simulink model "MSV_ublf"  (R2021a)
settings: Solver=ode4  StartTime=0.0  StopTime=10  FixedStep=0.001  MaxStep=0.01  RelTol=1e-3
model workspace (MAT data in the model file):
  EnableF = 1
  F_xyh = [10; 10; 1]
  GainKnownUncty = 1
  InputSat = [8591; 330.8; 839]
  InputSatOff = 1000
  Mmtx = [1  0  0; 0  1  0; 0  0  1]
  Temp = 0
  Test1 : Simulink.Parameter (value not decoded)
  boat_heading = 0
  boat_vel_x = 0
  boat_vel_y = 0
  earth_head = 2
  earth_x = 0
  earth_y = 2
  input_heading = 1
  input_x = 1
  input_y = 1
values from neighbouring files (symbols this model uses):
  Fval = [0 0 0]    [max_dist.m]    (also in test_ablf.m = [ ix iy iz ]; test_bs.m = [ ix iy iz ]; test_fxt.m = [ ix iy iz ]; test_max.m)
  LimStop = 0    [main.m]    (also in max_dist.m = 1)
libraries: dspmtrx3 x18, aerolibutil x5, simulink x1
(part 2 of 2)

== system MSV_ublf/MSV_w//uncertainty_BS/Gmatrix ==
  note: Set to 0 for G(x1) = [ 0 0 0]
  en : Inport
  x13 : Inport  Port=2
  Add g2 : Sum
  Cos : Trigonometry  Operator=cos
  Cos1 : Trigonometry  Operator=cos
  Gain : Gain  Gain=0.2
  Gain1 : Gain  Gain=0.36
  Gain2 : Gain  Gain=0.2
  Gain3 : Gain  Gain=0.36
  Matrix Concatenate : Concatenate  NumInputs=3  Mode=Multidimensional array
  Sin : Trigonometry
  Sin1 : Trigonometry
  Subtract g1 : Sum  Inputs=+-
  Switch : Switch  Criteria=u2 > Threshold
  g1 : Constant  Value=[0 0 0]'  VectorParams1D=off
  g3 : Constant  Value=0.18
  G(x1) : Outport
  wires:
  Gain2/1 -> Add g2/1
  Gain1/1 -> Subtract g1/2
  Add g2/1 -> Matrix Concatenate/2
  Sin1/1 -> Gain2/1
  x13/1 -> Cos1/1, Sin1/1, Sin/1, Cos/1
  Subtract g1/1 -> Matrix Concatenate/1
  Cos/1 -> Gain/1
  Gain/1 -> Subtract g1/1
  g3/1 -> Matrix Concatenate/3
  Sin/1 -> Gain1/1
  Gain3/1 -> Add g2/2
  Cos1/1 -> Gain3/1
  Switch/1 -> G(x1)/1
  Matrix Concatenate/1 -> Switch/1
  g1/1 -> Switch/3
  en/1 -> Switch/2

== system MSV_ublf/MSV_w//uncertainty_BS/J(η) // J (x1) ==
  note: SET = 1 FOR REVISED J(x1)
  note: Revised J(x1)
  note: Original from paper J(x1)
  note: SET = 0 FOR PAPER J(x1) [BELOW]
  Heading Angle : Inport
  Constant1 : Constant  Value=0
  Constant2 : Constant
  Constant3 : Constant  Value=0
  Constant4 : Constant
  Cos : Trigonometry  Operator=cos  OutputSignalType=real
  Cos1 : Trigonometry  Operator=cos  OutputSignalType=real
  Display : Display
  Gain1 : Gain  Gain=-1
  Gain2 : Gain  Gain=-1
  J select : Constant  Value=0
  Matrix Concatenate3 : Concatenate  NumInputs=3  Mode=Multidimensional array
  Matrix Concatenate4 : Concatenate  NumInputs=3  Mode=Multidimensional array  ConcatenateDimension=2
  Matrix Concatenate5 : Concatenate  NumInputs=3  Mode=Multidimensional array  ConcatenateDimension=2
  Matrix Concatenate6 : Concatenate  NumInputs=3  Mode=Multidimensional array  ConcatenateDimension=2
  Matrix Concatenate7 : Concatenate  NumInputs=3  Mode=Multidimensional array
  ROW 2 : Concatenate  NumInputs=3  Mode=Multidimensional array  ConcatenateDimension=2
  ROW1 : Concatenate  NumInputs=3  Mode=Multidimensional array  ConcatenateDimension=2
  ROW3 : Concatenate  NumInputs=3  Mode=Multidimensional array  ConcatenateDimension=2
  Sin : Trigonometry
  Sin1 : Trigonometry
  Switch : Switch  Criteria=u2 > Threshold
  J : Outport
  wires:
  ROW1/1 -> Matrix Concatenate3/1
  ROW 2/1 -> Matrix Concatenate3/2
  Constant2/1 -> ROW3/3
  Constant1/1 -> ROW 2/3, ROW3/2, ROW3/1, ROW1/3
  ROW3/1 -> Matrix Concatenate3/3
  Matrix Concatenate3/1 -> Switch/1
  Cos/1 -> ROW1/1, Gain1/1
  Sin/1 -> ROW1/2, ROW 2/1
  Gain1/1 -> ROW 2/2
  Cos1/1 -> Matrix Concatenate4/1, Matrix Concatenate5/2
  Matrix Concatenate6/1 -> Matrix Concatenate7/3
  Heading Angle/1 -> Cos1/1, Sin1/1, Sin/1, Cos/1
  Constant3/1 -> Matrix Concatenate4/3, Matrix Concatenate6/1, Matrix Concatenate6/2, Matrix Concatenate5/3
  Constant4/1 -> Matrix Concatenate6/3
  Matrix Concatenate5/1 -> Matrix Concatenate7/2
  Matrix Concatenate4/1 -> Matrix Concatenate7/1
  Sin1/1 -> Matrix Concatenate5/1, Gain2/1
  Switch/1 -> Display/1, J/1
  Matrix Concatenate7/1 -> Switch/3
  J select/1 -> Switch/2
  Gain2/1 -> Matrix Concatenate4/2

== system MSV_ublf/MSV_w//uncertainty_UBLF/Added Uncertainty ==
  Mdl : Inport
  Uct : Inport  Port=2
  Scope : Scope  NumInputPorts=3
  Selector : Selector  InputPortWidth=3  IndexOptions=Index vector (dialog)  Indices=1  OutputSizes=1
  Selector1 : Selector  InputPortWidth=3  IndexOptions=Index vector (dialog)  Indices=1  OutputSizes=1
  Selector2 : Selector  InputPortWidth=3  IndexOptions=Index vector (dialog)  Indices=2  OutputSizes=1
  Selector3 : Selector  InputPortWidth=3  IndexOptions=Index vector (dialog)  Indices=2  OutputSizes=1
  Selector4 : Selector  InputPortWidth=3  IndexOptions=Index vector (dialog)  Indices=3  OutputSizes=1
  Selector5 : Selector  InputPortWidth=3  IndexOptions=Index vector (dialog)  Indices=3  OutputSizes=1
  Vector Concatenate : Concatenate
  Vector Concatenate1 : Concatenate
  Vector Concatenate2 : Concatenate
  wires:
  Vector Concatenate/1 -> Scope/1
  Selector4/1 -> Vector Concatenate2/1  "mdl h"
  Selector/1 -> Vector Concatenate/1  "mdl x"
  Selector2/1 -> Vector Concatenate1/1  "mdl y"
  Vector Concatenate2/1 -> Scope/3
  Vector Concatenate1/1 -> Scope/2
  Selector1/1 -> Vector Concatenate/2  "uct x"
  Uct/1 -> Selector5/1, Selector3/1, Selector1/1
  Selector5/1 -> Vector Concatenate2/2  "uct h"
  Selector3/1 -> Vector Concatenate1/2  "uct y"
  Mdl/1 -> Selector4/1, Selector2/1, Selector/1

== system MSV_ublf/MSV_w//uncertainty_UBLF/Cmatrix ==
  x2 : Inport
  Add : Sum
  Constant : Constant  Value=0
  Gain : Gain  Gain=-24.6612
  Gain1 : Gain  Gain=25.8
  Gain2 : Gain  Gain=-25.8
  Gain3 : Gain  Gain=24.6612
  Gain4 : Gain  Gain=1.0948
  Matrix Concatenate3 : Concatenate  NumInputs=3  Mode=Multidimensional array
  Matrix Multiply : Product  Multiplication=Matrix(*)
  ROW 2 : Concatenate  NumInputs=3  Mode=Multidimensional array  ConcatenateDimension=2
  ROW1 : Concatenate  NumInputs=3  Mode=Multidimensional array  ConcatenateDimension=2
  ROW3 : Concatenate  NumInputs=3  Mode=Multidimensional array  ConcatenateDimension=2
  Row1[x2] : dspmtrx3/Submatrix  RowSpan=One row  RowStartMode=First  RowStartIndex=1  RowEndMode=Last  RowEndIndex=1  ColSpan=One column  ColStartMode=First  ColStartIndex=1  ColEndMode=Last  ColEndIndex=1
  Row2[x2] : dspmtrx3/Submatrix  RowSpan=One row  RowStartMode=Middle  RowStartIndex=1  RowEndMode=Last  RowEndIndex=1  ColSpan=One column  ColStartMode=First  ColStartIndex=1  ColEndMode=Last  ColEndIndex=1
  Row3[x2] : dspmtrx3/Submatrix  RowSpan=One row  RowStartMode=Last  RowStartIndex=1  RowEndMode=Last  RowEndIndex=1  ColSpan=One column  ColStartMode=First  ColStartIndex=1  ColEndMode=Last  ColEndIndex=1
  C(x2)x2 : Outport
  wires:
  ROW1/1 -> Matrix Concatenate3/1
  ROW 2/1 -> Matrix Concatenate3/2
  ROW3/1 -> Matrix Concatenate3/3
  Constant/1 -> ROW3/3, ROW 2/2, ROW 2/1, ROW1/2, ROW1/1
  Row1[x2]/1 -> Gain2/1, Gain1/1  "x_vel"
  Matrix Concatenate3/1 -> Matrix Multiply/1  "C(x2)"
  Gain/1 -> ROW1/3
  Gain1/1 -> ROW 2/3
  Gain2/1 -> ROW3/2
  Gain3/1 -> Add/1
  Row2[x2]/1 -> Gain/1, Gain3/1  "y_vel"
  Gain4/1 -> Add/2
  Add/1 -> ROW3/1
  Row3[x2]/1 -> Gain4/1  "ang_vel"
  x2/1 -> Matrix Multiply/2, Row3[x2]/1, Row1[x2]/1, Row2[x2]/1  "x2"
  Matrix Multiply/1 -> C(x2)x2/1

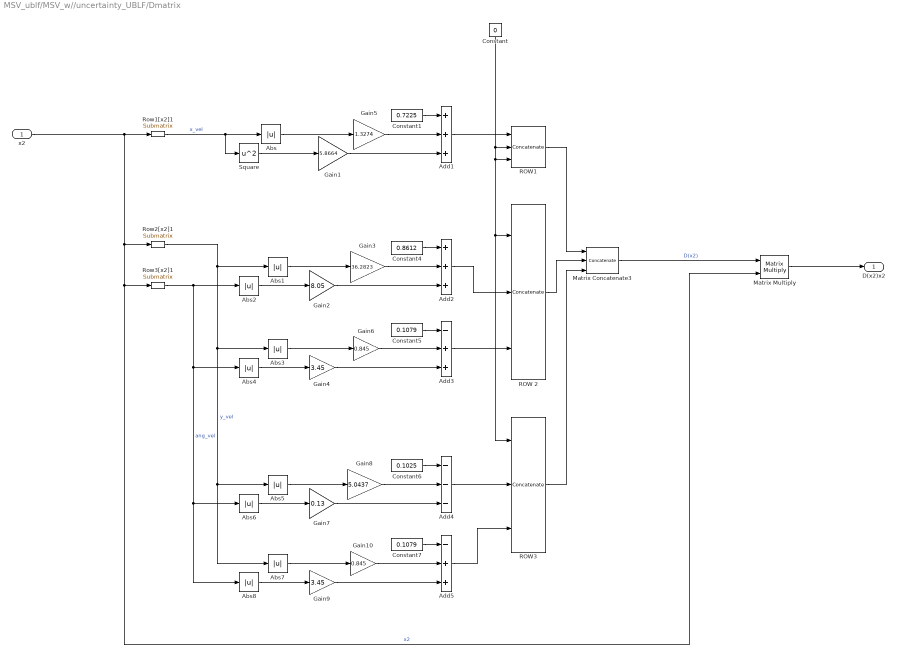
== system MSV_ublf/MSV_w//uncertainty_UBLF/Dmatrix ==
  x2 : Inport
  Abs{,1..8} (9 alike) : Abs
  Add1 : Sum  Inputs=+++
  Add2 : Sum  Inputs=+++
  Add3 : Sum  Inputs=-++
  Add4 : Sum  Inputs=---
  Add5 : Sum  Inputs=-++
  Constant : Constant  Value=0
  Constant1 : Constant  Value=0.7225
  Constant4 : Constant  Value=0.8612
  Constant5 : Constant  Value=0.1079
  Constant6 : Constant  Value=0.1025
  Constant7 : Constant  Value=0.1079
  Gain1 : Gain  Gain=5.8664
  Gain10 : Gain  Gain=0.845
  Gain2 : Gain  Gain=8.05
  Gain3 : Gain  Gain=36.2823
  Gain4 : Gain  Gain=3.45
  Gain5 : Gain  Gain=1.3274
  Gain6 : Gain  Gain=0.845
  Gain7 : Gain  Gain=0.13
  Gain8 : Gain  Gain=5.0437
  Gain9 : Gain  Gain=3.45
  Matrix Concatenate3 : Concatenate  NumInputs=3  Mode=Multidimensional array
  Matrix Multiply : Product  Multiplication=Matrix(*)
  ROW 2 : Concatenate  NumInputs=3  Mode=Multidimensional array  ConcatenateDimension=2
  ROW1 : Concatenate  NumInputs=3  Mode=Multidimensional array  ConcatenateDimension=2
  ROW3 : Concatenate  NumInputs=3  Mode=Multidimensional array  ConcatenateDimension=2
  Row1[x2]1 : dspmtrx3/Submatrix  RowSpan=One row  RowStartMode=First  RowStartIndex=1  RowEndMode=Last  RowEndIndex=1  ColSpan=One column  ColStartMode=First  ColStartIndex=1  ColEndMode=Last  ColEndIndex=1
  Row2[x2]1 : dspmtrx3/Submatrix  RowSpan=One row  RowStartMode=Middle  RowStartIndex=1  RowEndMode=Last  RowEndIndex=1  ColSpan=One column  ColStartMode=First  ColStartIndex=1  ColEndMode=Last  ColEndIndex=1
  Row3[x2]1 : dspmtrx3/Submatrix  RowSpan=One row  RowStartMode=Last  RowStartIndex=1  RowEndMode=Last  RowEndIndex=1  ColSpan=One column  ColStartMode=First  ColStartIndex=1  ColEndMode=Last  ColEndIndex=1
  Square : Math  Operator=square  SaturateOnIntegerOverflow=on
  D(x2)x2 : Outport
  wires:
  Constant/1 -> ROW 2/1, ROW3/1, ROW1/3, ROW1/2
  ROW3/1 -> Matrix Concatenate3/3
  ROW 2/1 -> Matrix Concatenate3/2
  ROW1/1 -> Matrix Concatenate3/1
  Constant1/1 -> Add1/1
  Gain5/1 -> Add1/2
  Gain1/1 -> Add1/3
  Abs/1 -> Gain5/1
  Square/1 -> Gain1/1
  Row1[x2]1/1 -> Abs/1, Square/1  "x_vel"
  Add1/1 -> ROW1/1
  Matrix Concatenate3/1 -> Matrix Multiply/1  "D(x2)"
  Abs1/1 -> Gain3/1
  Gain2/1 -> Add2/3
  Gain3/1 -> Add2/2
  Constant4/1 -> Add2/1
  Add2/1 -> ROW 2/2
  Abs2/1 -> Gain2/1
  Abs4/1 -> Gain4/1
  Constant5/1 -> Add3/1
  Gain6/1 -> Add3/2
  Gain4/1 -> Add3/3
  Abs3/1 -> Gain6/1
  Add3/1 -> ROW 2/3
  Row3[x2]1/1 -> Abs8/1, Abs6/1, Abs4/1, Abs2/1  "ang_vel"
  Abs7/1 -> Gain10/1
  Gain9/1 -> Add5/3
  Gain10/1 -> Add5/2
  Constant7/1 -> Add5/1
  Abs8/1 -> Gain9/1
  Row2[x2]1/1 -> Abs7/1, Abs5/1, Abs3/1, Abs1/1  "y_vel"
  Abs6/1 -> Gain7/1
  Constant6/1 -> Add4/1
  Gain8/1 -> Add4/2
  Gain7/1 -> Add4/3
  Abs5/1 -> Gain8/1
  Add4/1 -> ROW3/2
  Add5/1 -> ROW3/3
  x2/1 -> Matrix Multiply/2, Row3[x2]1/1, Row2[x2]1/1, Row1[x2]1/1  "x2"
  Matrix Multiply/1 -> D(x2)x2/1

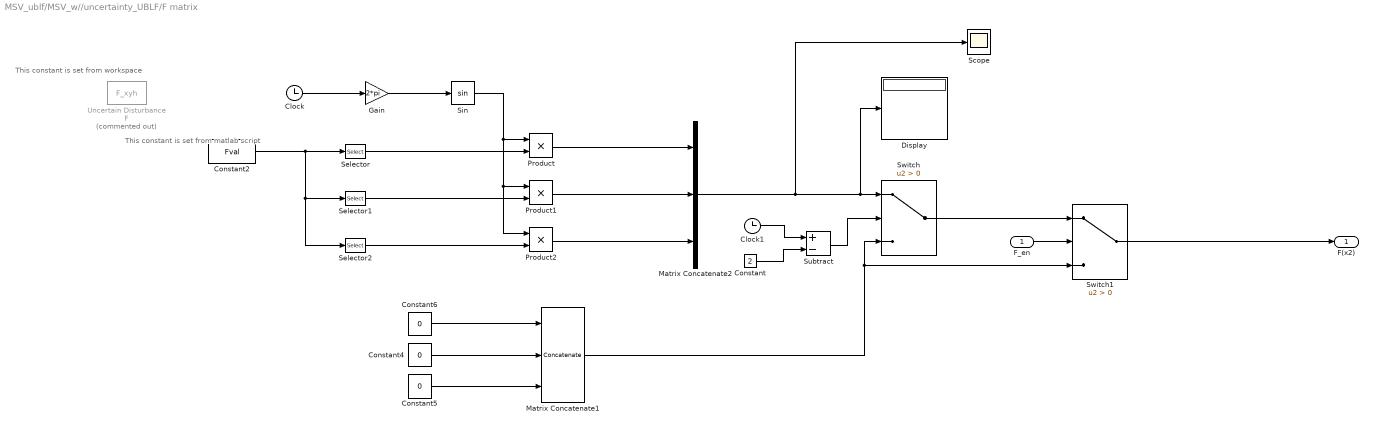
== system MSV_ublf/MSV_w//uncertainty_UBLF/F matrix ==
  note: This constant is set from matlab script
  note: This constant is set from workspace
  F_en : Inport
  Clock : Clock
  Clock1 : Clock
  Constant : Constant  Value=2
  Constant2 : Constant  Value=Fval
  Constant4 : Constant  Value=0
  Constant5 : Constant  Value=0
  Constant6 : Constant  Value=0
  Display : Display
  Gain : Gain  Gain=2*pi
  Matrix Concatenate1 : Concatenate  NumInputs=3  Mode=Multidimensional array
  Matrix Concatenate2 : Concatenate  NumInputs=3  Mode=Multidimensional array
  Product : Product
  Product1 : Product
  Product2 : Product
  Scope : Scope
  Selector : Selector  InputPortWidth=3  IndexOptions=Index vector (dialog)  Indices=1  OutputSizes=1
  Selector1 : Selector  InputPortWidth=3  IndexOptions=Index vector (dialog)  Indices=2  OutputSizes=1
  Selector2 : Selector  InputPortWidth=3  IndexOptions=Index vector (dialog)  Indices=3  OutputSizes=1
  Sin : Trigonometry
  Subtract : Sum  Inputs=+-
  Switch : Switch  Criteria=u2 > Threshold
  Switch1 : Switch  Criteria=u2 > Threshold
  Uncertain Disturbance F : Constant  Commented=on  Value=F_xyh
  F(x2) : Outport
  wires:
  F_en/1 -> Switch1/2
  Switch1/1 -> F(x2)/1
  Constant5/1 -> Matrix Concatenate1/3
  Constant4/1 -> Matrix Concatenate1/2
  Constant6/1 -> Matrix Concatenate1/1
  Matrix Concatenate1/1 -> Switch1/3, Switch/3
  Matrix Concatenate2/1 -> Scope/1, Display/1, Switch/1
  Clock1/1 -> Subtract/1
  Constant/1 -> Subtract/2
  Subtract/1 -> Switch/2
  Switch/1 -> Switch1/1
  Product/1 -> Matrix Concatenate2/1
  Product2/1 -> Matrix Concatenate2/3
  Product1/1 -> Matrix Concatenate2/2
  Sin/1 -> Product1/1, Product2/1, Product/1
  Selector/1 -> Product/2
  Selector1/1 -> Product1/2
  Selector2/1 -> Product2/2
  Gain/1 -> Sin/1
  Clock/1 -> Gain/1
  Constant2/1 -> Selector2/1, Selector1/1, Selector/1

== system MSV_ublf/MSV_w//uncertainty_UBLF/Gmatrix ==
  note: Set to 0 for G(x1) = [ 0 0 0]
  en : Inport
  x13 : Inport  Port=2
  Add g2 : Sum
  Cos : Trigonometry  Operator=cos
  Cos1 : Trigonometry  Operator=cos
  Gain : Gain  Gain=0.2
  Gain1 : Gain  Gain=0.36
  Gain2 : Gain  Gain=0.2
  Gain3 : Gain  Gain=0.36
  Matrix Concatenate : Concatenate  NumInputs=3  Mode=Multidimensional array
  Sin : Trigonometry
  Sin1 : Trigonometry
  Subtract g1 : Sum  Inputs=+-
  Switch : Switch  Criteria=u2 > Threshold
  g1 : Constant  Value=[0 0 0]'  VectorParams1D=off
  g3 : Constant  Value=0.18
  G(x1) : Outport
  wires:
  Gain2/1 -> Add g2/1
  Gain1/1 -> Subtract g1/2
  Add g2/1 -> Matrix Concatenate/2
  Sin1/1 -> Gain2/1
  x13/1 -> Cos1/1, Sin1/1, Sin/1, Cos/1
  Subtract g1/1 -> Matrix Concatenate/1
  Cos/1 -> Gain/1
  Gain/1 -> Subtract g1/1
  g3/1 -> Matrix Concatenate/3
  Sin/1 -> Gain1/1
  Gain3/1 -> Add g2/2
  Cos1/1 -> Gain3/1
  Switch/1 -> G(x1)/1
  Matrix Concatenate/1 -> Switch/1
  g1/1 -> Switch/3
  en/1 -> Switch/2

== system MSV_ublf/MSV_w//uncertainty_UBLF/J(η) // J (x1) ==
  note: SET = 1 FOR REVISED J(x1)
  note: Revised J(x1)
  note: Original from paper J(x1)
  note: SET = 0 FOR PAPER J(x1) [BELOW]
  Heading Angle : Inport
  Constant1 : Constant  Value=0
  Constant2 : Constant
  Constant3 : Constant  Value=0
  Constant4 : Constant
  Cos : Trigonometry  Operator=cos  OutputSignalType=real
  Cos1 : Trigonometry  Operator=cos  OutputSignalType=real
  Display : Display
  Gain1 : Gain  Gain=-1
  Gain2 : Gain  Gain=-1
  J select : Constant  Value=0
  Matrix Concatenate3 : Concatenate  NumInputs=3  Mode=Multidimensional array
  Matrix Concatenate4 : Concatenate  NumInputs=3  Mode=Multidimensional array  ConcatenateDimension=2
  Matrix Concatenate5 : Concatenate  NumInputs=3  Mode=Multidimensional array  ConcatenateDimension=2
  Matrix Concatenate6 : Concatenate  NumInputs=3  Mode=Multidimensional array  ConcatenateDimension=2
  Matrix Concatenate7 : Concatenate  NumInputs=3  Mode=Multidimensional array
  ROW 2 : Concatenate  NumInputs=3  Mode=Multidimensional array  ConcatenateDimension=2
  ROW1 : Concatenate  NumInputs=3  Mode=Multidimensional array  ConcatenateDimension=2
  ROW3 : Concatenate  NumInputs=3  Mode=Multidimensional array  ConcatenateDimension=2
  Sin : Trigonometry
  Sin1 : Trigonometry
  Switch : Switch  Criteria=u2 > Threshold
  J : Outport
  wires:
  ROW1/1 -> Matrix Concatenate3/1
  ROW 2/1 -> Matrix Concatenate3/2
  Constant2/1 -> ROW3/3
  Constant1/1 -> ROW 2/3, ROW3/2, ROW3/1, ROW1/3
  ROW3/1 -> Matrix Concatenate3/3
  Matrix Concatenate3/1 -> Switch/1
  Cos/1 -> ROW1/1, Gain1/1
  Sin/1 -> ROW1/2, ROW 2/1
  Gain1/1 -> ROW 2/2
  Cos1/1 -> Matrix Concatenate4/1, Matrix Concatenate5/2
  Matrix Concatenate6/1 -> Matrix Concatenate7/3
  Heading Angle/1 -> Cos1/1, Sin1/1, Sin/1, Cos/1
  Constant3/1 -> Matrix Concatenate4/3, Matrix Concatenate6/1, Matrix Concatenate6/2, Matrix Concatenate5/3
  Constant4/1 -> Matrix Concatenate6/3
  Matrix Concatenate5/1 -> Matrix Concatenate7/2
  Matrix Concatenate4/1 -> Matrix Concatenate7/1
  Sin1/1 -> Matrix Concatenate5/1, Gain2/1
  Switch/1 -> Display/1, J/1
  Matrix Concatenate7/1 -> Switch/3
  J select/1 -> Switch/2
  Gain2/1 -> Matrix Concatenate4/2

== matlab function MSV_ublf/Backstepping Control/MATLAB Function ==
  settings: updateMethod=DISCRETE
  data: CDG input; u output; x_Err output; y_Err output; h_Err output; M input; J input; X1 input; X2 input; X1d input; unused input; unused1 input size=1; test1 output; test2 output
function [u, x_Err, y_Err, h_Err, test1, test2] =  fcn( CDG, M, J ,X1, X2, X1d, ~, ~)
    
    tstep   = 0.001;
    
    persistent last_alpha1 
    if isempty(last_alpha1) 
        last_alpha1=X2;
    end
    
    persistent last_X1d 
    if isempty(last_X1d) 
        last_X1d=X1d;
    end
    
    X1d_dot = (X1d - last_X1d)/tstep;
    last_X1d = X1d;

    JT      = J';    % Transpose jacobian

    
    % Set Gain Values
    K1      = 30 ; % 100*[ 0.01 ; 0.01 ; 0.01 ];           % Gains used with ALPHA1    ### NOTE SET MUCH HIGHER THAN VALUES IN PAPER ####
    K2      = 200; %5*[ 20 0 0 ; 0 20 0 ; 0 0 20 ];     % Gains used with u          ### NOTE SET MUCH HIGHER THAN VALUES IN PAPER ####
    

% ### STEP 1 ###
    
    Z1      = X1 - X1d;          % Z1 position/hdg error
    
    %ALPHA 1

    ALPHA1  = JT*(X1d_dot - Z1.*K1 );
    
    A1_dot = (ALPHA1-last_alpha1)/tstep;
    last_alpha1 = ALPHA1;
    
% ### STEP 2 ###

    Z2      = X2 - ALPHA1;  % Z2 velocity error
    CTRL    = -CDG - J*Z1 - K2.*Z2 + M*A1_dot;
    
% Function Outputs

u       = CTRL;
x_Err   = 0;
y_Err   = 0;
h_Err   = 0;
test1   = 0;
test2   = Z1;

== matlab function MSV_ublf/FxT uBLF_v1.1/SymUBLF1 ==
  settings: updateMethod=DISCRETE
  data: F2 input; G2 input; G1 input; X1 input; X2 input; Xd input; unused input; unused1 input; u output; xErr output; yErr output; hErr output; test1 output
function [u,xErr, yErr, hErr, test1 ] = fcn(F2, G2, G1, X1, X2, Xd, ~, ~)

    %Simulation settings
    tstep = 0.001;
    
    % Set persistent variables for derivatives
    persistent last_x1d
    if isempty (last_x1d)
        last_x1d = Xd;
    end
    
    persistent last_A1
    if isempty(last_A1)
        last_A1 = X2;
    end
    
    % K (3x1) Barrier limits
    K       = 5*[ 0.005
                0.005
                0.005 ]; 

    % fixed time parameters (a/b maybe should be vectors?)
      
    a1      = 5;
    b1      = 1;
    a2      = 5;
    b2      = 1;

    eps10   = 0.00001;
    eps20   = 0.00001;
    
    eps1    = 0.00008;
    eps2    = 0.00001;

% ### STEP 1 ####

    % Z1 (3x1) - Position error
    Z1      = X1 - Xd;
    
    % ETA (3x1)
    ETA     = ((K.^2).*Z1) ./ ( (K.^2)-(Z1.^2)); 
    nETA    = norm(ETA); %mETA    = sqrt(sum(ETA.^2)); % magnitude of ETA vector for S1 switched term ¦ changed to norm(ETA) ?
    
    % OMEGA (3x1)
    OMEGA   = ( (K.^2).*( (K.^2)+(Z1.^2) ) ) ./ ( ( (K.^2)-(Z1.^2) ).^2 ) ;

    % Switched Term 1st step S1
    if nETA < eps10
        %test%S1 = ( (ETA.^2).^(3/4)); 
        S1 = (5/4)*(ETA' * ETA)*((eps10^2)^(-1/4)) +  (-1/4)*((ETA' * ETA)^2)*((eps10^2)^(-5/4)) ;
    else
       S1 = ( (ETA' * ETA)^(3/4));        
    end
    
    % X1 derivative used in ALPHA1
    Xd_dot = (Xd - last_x1d)/tstep;
    last_x1d = Xd;
    
    % Calculate ALPHA1 virtual control for step 2
    ALPHA1_HAT  = -(OMEGA.*Xd_dot) +  ( (0.5^(3/4))*a1 )*( (ETA/(ETA' * ETA))*S1 ) + ((0.5^2)*b1)*((ETA*(ETA' * ETA))) ;
    ALPHA1_BAR  = diag([1/OMEGA(1) 1/OMEGA(2) 1/OMEGA(3)])*ALPHA1_HAT;
    nA1B        = norm(ALPHA1_BAR);
    ETA_OMEGA   = ETA .* OMEGA;
    nETA_OMEGA  = norm(ETA_OMEGA);
    g1          = inv(G1);
    
    ALPHA1      = -g1 * (  (ETA_OMEGA*((nA1B)^2) ) / ( sqrt( ( (nETA_OMEGA)^2 ) * ( (nA1B)^2 ) + eps1^2 ) )  );
    
% ### STEP 2 ###

    %Z2 = X2 - ALPHA1
    Z2      = X2 - ALPHA1;
    nZ2     = norm(Z2);   % norm of vector Z2 used to select S2 term below
    
    % Switched Term 2nd step S2
    if nZ2 < eps20
        %test S2 = ( (Z2.^2).^(3/4));
        S2 = (5/4)*(Z2' * Z2)*((eps20^2)^(-1/4)) +  (-1/4)*((Z2' * Z2).^2)*((eps20^2)^(-5/4)) ;
    else
       S2 = ( (Z2' * Z2)^(3/4));        
    end
    
    % ALPHA1 derivative used in ALPHA2_HAT
    A1_dot = (ALPHA1 - last_A1)/tstep;
    last_A1 = ALPHA1;    
    
    % Calculate control signal
    AH2_A       = ( (0.5^(3/4))*a2 )*( (Z2 / (Z2' * Z2))*S2 );
    AH2_B       = ( (0.5^2)*b2) * ((Z2*(Z2' * Z2)           ));
    ALPHA2_HAT  = ( -(A1_dot) + AH2_A + AH2_B );
    g2          = inv(G2);
    CTRL        = -g2 * ( (Z2 .* (ALPHA2_HAT.^2)) ./ ( sqrt (((Z2.^2).*(ALPHA2_HAT.^2) + eps2^2)) ) + (G1 * ETA_OMEGA) +F2 );      

%Function outputs
xErr    = [Z1(1) ; K(1) ; -K(1)];   % error and BLF limits
yErr    = [Z1(2) ; K(2) ; -K(2)];   % error and BLF limits
hErr    = [Z1(3) ; K(3) ; -K(3)];   % error and BLF limits
test1   = 0;                        % test output
u       = CTRL;


%%[2022.02.23.Wed] Changed Functions from v1.2(correcting for elementwise to matrix functions)

%     % Switched Term 1st step S1
%     if mETA < eps10
%         %test%S1 = ( (ETA.^2).^(3/4)); 
%         S1 = (5/4)*(ETA.^2)*((eps10^2)^(-1/4)) +  (-1/4)*((ETA.^2).^2)*((eps10^2)^(-5/4)) ;
%     else
%        S1 = ( (ETA.^2).^(3/4));        
%     end

%     % Calculate ALPHA1 virtual control for step 2
%     ALPHA1_HAT  = -(OMEGA.*Xd_dot) + ( ((0.5^(3/4)).*a1).*((ETA ./ (ETA.^2)).*S1) ) + ( ((0.5^2).*b1).*((ETA.*(ETA.^2))) );
%     ALPHA1_BAR  = diag([1/OMEGA(1) 1/OMEGA(2) 1/OMEGA(3)])*ALPHA1_HAT;
%     nA1B        = norm(ALPHA1_BAR);
%     ETA_OMEGA   = ETA .* OMEGA;
%     nETA_OMEGA  = norm(ETA_OMEGA);
%     g1          = inv(G1);

    % wrong sqrt in denom of ALPHA1 below
%   ALPHA1      = -g1 * (( ETA_OMEGA*((nA1B)^2) ) ./ (sqrt( (nETA_OMEGA)^2)*((nA1B)^2) + eps1^2  ));

== matlab function MSV_ublf/FxT uBLF_v1.4/SymUBLF1 ==
  settings: updateMethod=DISCRETE
  data: F2 input; G2 input; G1 input; X1 input; X2 input; Xd input; unused input; unused1 input; u output; xErr output; yErr output; hErr output; test1 output
function [u,xErr, yErr, hErr, test1 ] = fcn(F2, G2, G1, X1, X2, Xd, ~, ~)

    %Simulation settings
    tstep = 0.001;
    
    % Set persistent variables for derivatives
    persistent last_x1d
    if isempty (last_x1d)
        last_x1d = Xd;
    end
    
    persistent last_A1
    if isempty(last_A1)
        last_A1 = X2;
    end
    
    % K (3x1) Barrier limits
    K       = 5*[ 0.005
                0.005
                0.005 ]; 

    % fixed time parameters (a/b maybe should be vectors?)
      
    a1      = 5;
    b1      = 1;
    a2      = 5;
    b2      = 1;

    eps10   = 0.00001;
    eps20   = 0.00001;
    
    eps1    = 0.00008;
    eps2    = 0.00001;

% ### STEP 1 ####

    % Z1 (3x1) - Position error
    Z1      = X1 - Xd;
    
    % ETA (3x1)
    ETA     = ((K.^2).*Z1) ./ ( (K.^2)-(Z1.^2)); 
    nETA    = norm(ETA); %mETA    = sqrt(sum(ETA.^2)); % magnitude of ETA vector for S1 switched term ¦ changed to norm(ETA) ?
    
    % OMEGA (3x1)
    OMEGA   = ( (K.^2).*( (K.^2)+(Z1.^2) ) ) ./ ( ( (K.^2)-(Z1.^2) ).^2 ) ;

    % Switched Term 1st step S1
    if nETA < eps10
        %test%S1 = ( (ETA.^2).^(3/4)); 
        S1 = (5/4)*(ETA' * ETA)*((eps10^2)^(-1/4)) +  (-1/4)*((ETA' * ETA)^2)*((eps10^2)^(-5/4)) ;
    else
       S1 = ( (ETA' * ETA)^(3/4));        
    end
    
    % X1 derivative used in ALPHA1
    Xd_dot = (Xd - last_x1d)/tstep;
    last_x1d = Xd;
    
    % Calculate ALPHA1 virtual control for step 2
    ALPHA1_HAT  = -(OMEGA.*Xd_dot) +  ( (0.5^(3/4))*a1 )*( (ETA/(ETA' * ETA))*S1 ) + ((0.5^2)*b1)*((ETA*(ETA' * ETA))) ;
    ALPHA1_BAR  = diag([1/OMEGA(1) 1/OMEGA(2) 1/OMEGA(3)])*ALPHA1_HAT;
    nA1B        = norm(ALPHA1_BAR);
    ETA_OMEGA   = ETA .* OMEGA;
    nETA_OMEGA  = norm(ETA_OMEGA);
    g1          = inv(G1);
    
    ALPHA1      = -g1 * (  (ETA_OMEGA*((nA1B)^2) ) / ( sqrt( ( (nETA_OMEGA)^2 ) * ( (nA1B)^2 ) + eps1^2 ) )  );
    
% ### STEP 2 ###

    %Z2 = X2 - ALPHA1
    Z2      = X2 - ALPHA1;
    nZ2     = norm(Z2);   % norm of vector Z2 used to select S2 term below
    
    % Switched Term 2nd step S2
    if nZ2 < eps20
        %test S2 = ( (Z2.^2).^(3/4));
        S2 = (5/4)*(Z2' * Z2)*((eps20^2)^(-1/4)) +  (-1/4)*((Z2' * Z2).^2)*((eps20^2)^(-5/4)) ;
    else
       S2 = ( (Z2' * Z2)^(3/4));        
    end
    
    % ALPHA1 derivative used in ALPHA2_HAT
    A1_dot = (ALPHA1 - last_A1)/tstep;
    last_A1 = ALPHA1;    
    
    % Calculate control signal
    AH2_A       = ( (0.5^(3/4))*a2 )*( (Z2 / (Z2' * Z2))*S2 );
    AH2_B       = ( (0.5^2)*b2) * ((Z2*(Z2' * Z2)           ));
    ALPHA2_HAT  = ( -(A1_dot) + AH2_A + AH2_B );
    g2          = inv(G2);
    CTRL        = -g2 * ( (Z2 .* (ALPHA2_HAT.^2)) ./ ( sqrt (((Z2.^2).*(ALPHA2_HAT.^2) + eps2^2)) ) + (G1 * ETA_OMEGA) +F2 );      

%Function outputs
xErr    = [Z1(1) ; K(1) ; -K(1)];   % error and BLF limits
yErr    = [Z1(2) ; K(2) ; -K(2)];   % error and BLF limits
hErr    = [Z1(3) ; K(3) ; -K(3)];   % error and BLF limits
test1   = 0;                        % test output
u       = CTRL;


%%[2022.02.23.Wed] Changed Functions from v1.2(correcting for elementwise to matrix functions)

%     % Switched Term 1st step S1
%     if mETA < eps10
%         %test%S1 = ( (ETA.^2).^(3/4)); 
%         S1 = (5/4)*(ETA.^2)*((eps10^2)^(-1/4)) +  (-1/4)*((ETA.^2).^2)*((eps10^2)^(-5/4)) ;
%     else
%        S1 = ( (ETA.^2).^(3/4));        
%     end

%     % Calculate ALPHA1 virtual control for step 2
%     ALPHA1_HAT  = -(OMEGA.*Xd_dot) + ( ((0.5^(3/4)).*a1).*((ETA ./ (ETA.^2)).*S1) ) + ( ((0.5^2).*b1).*((ETA.*(ETA.^2))) );
%     ALPHA1_BAR  = diag([1/OMEGA(1) 1/OMEGA(2) 1/OMEGA(3)])*ALPHA1_HAT;
%     nA1B        = norm(ALPHA1_BAR);
%     ETA_OMEGA   = ETA .* OMEGA;
%     nETA_OMEGA  = norm(ETA_OMEGA);
%     g1          = inv(G1);

    % wrong sqrt in denom of ALPHA1 below
%   ALPHA1      = -g1 * (( ETA_OMEGA*((nA1B)^2) ) ./ (sqrt( (nETA_OMEGA)^2)*((nA1B)^2) + eps1^2  ));

== matlab function MSV_ublf/FxT uBLF_v1.1/UBLF ==
  settings: updateMethod=DISCRETE
  data: F2 input; G2 input; G1 input; X1 input; X2 input; Xd input; unused input; unused1 input; u output; xErr output; yErr output; hErr output; test1 output; test2 output
function [u,xErr, yErr, hErr, test1, test2 ] = fcn(F2, G2, G1, X1, X2, Xd, ~, ~)

    %Simulation settings
    tstep = 0.001;
    
    % Set persistent variables for derivatives
    persistent last_x1d
    if isempty (last_x1d)
        last_x1d = Xd;
    end
    
    persistent last_A1
    if isempty(last_A1)
        last_A1 = X2;
    end
    
    % Barrier limits
    % Lower Limit (-KL)
    KL      = 1*[   0.008
                    0.005
                    0.006 ];       
    % Higher/Upper Limit (KH)
    KH      = 1*[   0.016
                    0.015
                    0.011 ]; 
    % fixed time parameterS
      
    a1      = 2*5;
    b1      = 30;
    a2      = 2*5;
    b2      = 30;

    eps10   = 0.0001;
    eps20   = 0.0001;
    
    eps1    = 0.00005;
    eps2    = eps1;
    
    kpa1 = min(a1,a2);
    kpa2 = min(b1,b2);
    
    tmax = 5.867/kpa1 + 1/kpa2;

% ### STEP 1 ####

    % Z1 (3x1) - Position error
    Z1      = X1 - Xd;
    
    % ETA (3x1)
    ETA     = ( (KH .* KL).*Z1 ) ./ ( (KH - Z1) .* (KL + Z1) ) ; 
    nETA    = norm(ETA); %mETA    = sqrt(sum(ETA.^2)); % magnitude of ETA vector for S1 switched term ¦ changed to norm(ETA) ?
    
    % OMEGA (3x1)
    OMEGA   = ( KH .* KL .*(KH .* KL + Z1.^2 ) ) ./ ( (KH - Z1).^2  .* (KL + Z1).^2 ) ;

    % Switched Term 1st step S1
    if nETA < eps10
        %test%S1 = ( (ETA.^2).^(3/4)); 
        S1 = (5/4)*(ETA' * ETA)*((eps10^2)^(-1/4)) +  (-1/4)*((ETA' * ETA)^2)*((eps10^2)^(-5/4)) ;
    else
       S1 = ( (ETA' * ETA)^(3/4));        
    end
    
    % X1 derivative used in ALPHA1
    Xd_dot = (Xd - last_x1d)/tstep;
    last_x1d = Xd;
    
    % Calculate ALPHA1 virtual control for step 2
    ALPHA1_HAT  = -(OMEGA.*Xd_dot) +  ( (0.5^(3/4))*a1 )*( (ETA/(ETA' * ETA))*S1 ) + ((0.5^2)*b1)*((ETA*(ETA' * ETA))) ;
    ALPHA1_BAR  = diag([1/OMEGA(1) 1/OMEGA(2) 1/OMEGA(3)])*ALPHA1_HAT;
    nA1B        = norm(ALPHA1_BAR);
    ETA_OMEGA   = ETA .* OMEGA;
    nETA_OMEGA  = norm(ETA_OMEGA);
    g1          = G1';
    
    ALPHA1      = -g1 * (  (ETA_OMEGA*((nA1B)^2) ) / ( sqrt( ( (nETA_OMEGA)^2 ) * ( (nA1B)^2 ) + eps1^2 ) )  );
    
% ### STEP 2 ###

    %Z2 = X2 - ALPHA1
    Z2      = X2 - ALPHA1;
    nZ2     = norm(Z2);   % norm of vector Z2 used to select S2 term below
    
    % Switched Term 2nd step S2
    if nZ2 < eps20
        %test S2 = ( (Z2.^2).^(3/4));
        S2 = (5/4)*(Z2' * Z2)*((eps20^2)^(-1/4)) +  (-1/4)*((Z2' * Z2).^2)*((eps20^2)^(-5/4)) ;
    else
       S2 = ( (Z2' * Z2)^(3/4));        
    end
    
    % ALPHA1 derivative used in ALPHA2_HAT
    A1_dot = (ALPHA1 - last_A1)/tstep;
    last_A1 = ALPHA1;    
    
    % Calculate control signal
    AH2_A       = ( (0.5^(3/4))*a2 )*( (Z2 / (Z2' * Z2))*S2 );
    AH2_B       = ( (0.5^2)*b2) * ((Z2*(Z2' * Z2)           ));
    ALPHA2_HAT  = ( -(A1_dot) + AH2_A + AH2_B );
    g2          = inv(G2);
    CTRL        = -g2 * ( (Z2 .* (ALPHA2_HAT.^2)) ./ ( sqrt (((Z2.^2).*(ALPHA2_HAT.^2) + eps2^2)) ) + (Z2/(Z2'*Z2))*ETA_OMEGA'*g1*Z2 + F2 );
%   CTRL        = -g2 * ( (Z2 .* (ALPHA2_HAT.^2)) ./ ( sqrt (((Z2.^2).*(ALPHA2_HAT.^2) + eps2^2)) ) + (G1 * ETA_OMEGA) +F2 );  

%Function outputs
xErr    = [Z1(1) ; KH(1) ; -KL(1)];   % error and BLF limits
yErr    = [Z1(2) ; KH(2) ; -KL(2)];   % error and BLF limits
hErr    = [Z1(3) ; KH(3) ; -KL(3)];   % error and BLF limits
test1   = Z1 ;                        % test output
test2   = [tmax, a1, a2, b1, b2, eps1, eps2, eps10, eps20]';
u       = CTRL;


%%[2022.02.23.Wed] Changed Functions from v1.2(correcting for elementwise to matrix functions)

%     % Switched Term 1st step S1
%     if mETA < eps10
%         %test%S1 = ( (ETA.^2).^(3/4)); 
%         S1 = (5/4)*(ETA.^2)*((eps10^2)^(-1/4)) +  (-1/4)*((ETA.^2).^2)*((eps10^2)^(-5/4)) ;
%     else
%        S1 = ( (ETA.^2).^(3/4));        
%     end

%     % Calculate ALPHA1 virtual control for step 2
%     ALPHA1_HAT  = -(OMEGA.*Xd_dot) + ( ((0.5^(3/4)).*a1).*((ETA ./ (ETA.^2)).*S1) ) + ( ((0.5^2).*b1).*((ETA.*(ETA.^2))) );
%     ALPHA1_BAR  = diag([1/OMEGA(1) 1/OMEGA(2) 1/OMEGA(3)])*ALPHA1_HAT;
%     nA1B        = norm(ALPHA1_BAR);
%     ETA_OMEGA   = ETA .* OMEGA;
%     nETA_OMEGA  = norm(ETA_OMEGA);
%     g1          = inv(G1);

    % wrong sqrt in denom of ALPHA1 below
%   ALPHA1      = -g1 * (( ETA_OMEGA*((nA1B)^2) ) ./ (sqrt( (nETA_OMEGA)^2)*((nA1B)^2) + eps1^2  ));

== matlab function MSV_ublf/limits stop/MATLAB Function ==
  data: Z1 input; rtn output; en input
function rtn = fcn(Z1, en)
    y = 0 ;
    if en == 1

        %Limits
        z1_h = 0.016;           %   KA      = [ 0.008 ; 0.005 ; 0.006 ];    % Negative Barrier limit (as in paper)
        z1_l = 0.008;           %   KB      = [ 0.016 ; 0.015 ; 0.011 ];    % Positive Barrier limit (as in paper)
        z2_h = 0.015;
        z2_l = 0.005;
        z3_h = 0.011;
        z3_l = 0.006;

        if Z1(1) < -(z1_l) || Z1(1) > z1_h
            y = 1;        
        end

        if Z1(2) < -(z2_l) || Z1(2) > z2_h
            y = 1;        
        end

        if Z1(3) < -(z3_l) || Z1(3) > z3_h
            y = 1;        
        end
        
        if y ==1
            error('Error is beyond limits');
        end
    
    end

rtn = y;

== matlab function MSV_ublf/FxT uBLF_v1.4/UBLF ==
  settings: updateMethod=DISCRETE
  data: F2 input; G2 input; G1 input; X1 input; X2 input; Xd input; unused input; unused1 input; u output; xErr output; yErr output; hErr output; test1 output; test2 output
function [u,xErr, yErr, hErr, test1, test2 ] = fcn(F2, G2, G1, X1, X2, Xd, ~, ~)

    %Simulation settings
    tstep = 0.001;
    
    % Set persistent variables for derivatives
    persistent last_x1d
    if isempty (last_x1d)
        last_x1d = Xd;
    end
    
    persistent last_A1
    if isempty(last_A1)
        last_A1 = X2;
    end
    
    % Barrier limits
    % Lower Limit (-KL)
    KL      = 1*[   0.008
                    0.005
                    0.006 ];       
    % Higher/Upper Limit (KH)
    KH      = 1*[   0.016
                    0.015
                    0.011 ]; 
    % fixed time parameterS
      
    a1      = 2*5;
    b1      = 30;
    a2      = 2*5;
    b2      = 30;

    eps10   = 0.0001;
    eps20   = 0.0001;
    
    eps1    = 0.00005;
    eps2    = eps1;
    
    kpa1 = min(a1,a2);
    kpa2 = min(b1,b2);
    
    tmax = 5.867/kpa1 + 1/kpa2;

% ### STEP 1 ####

    % Z1 (3x1) - Position error
    Z1      = X1 - Xd;
    
    % ETA (3x1)
    ETA     = ( (KH .* KL).*Z1 ) ./ ( (KH - Z1) .* (KL + Z1) ) ; 
    nETA    = norm(ETA); %mETA    = sqrt(sum(ETA.^2)); % magnitude of ETA vector for S1 switched term ¦ changed to norm(ETA) ?
    
    % OMEGA (3x1)
    OMEGA   = ( KH .* KL .*(KH .* KL + Z1.^2 ) ) ./ ( (KH - Z1).^2  .* (KL + Z1).^2 ) ;

    % Switched Term 1st step S1
    if nETA < eps10
        %test%S1 = ( (ETA.^2).^(3/4)); 
        S1 = (5/4)*(ETA' * ETA)*((eps10^2)^(-1/4)) +  (-1/4)*((ETA' * ETA)^2)*((eps10^2)^(-5/4)) ;
    else
       S1 = ( (ETA' * ETA)^(3/4));        
    end
    
    % X1 derivative used in ALPHA1
    Xd_dot = (Xd - last_x1d)/tstep;
    last_x1d = Xd;
    
    % Calculate ALPHA1 virtual control for step 2
    ALPHA1_HAT  = -(OMEGA.*Xd_dot) +  ( (0.5^(3/4))*a1 )*( (ETA/(ETA' * ETA))*S1 ) + ((0.5^2)*b1)*((ETA*(ETA' * ETA))) ;
    ALPHA1_BAR  = diag([1/OMEGA(1) 1/OMEGA(2) 1/OMEGA(3)])*ALPHA1_HAT;
    nA1B        = norm(ALPHA1_BAR);
    ETA_OMEGA   = ETA .* OMEGA;
    nETA_OMEGA  = norm(ETA_OMEGA);
    g1          = G1';
    
    ALPHA1      = -g1 * (  (ETA_OMEGA*((nA1B)^2) ) / ( sqrt( ( (nETA_OMEGA)^2 ) * ( (nA1B)^2 ) + eps1^2 ) )  );
    
% ### STEP 2 ###

    %Z2 = X2 - ALPHA1
    Z2      = X2 - ALPHA1;
    nZ2     = norm(Z2);   % norm of vector Z2 used to select S2 term below
    
    % Switched Term 2nd step S2
    if nZ2 < eps20
        %test S2 = ( (Z2.^2).^(3/4));
        S2 = (5/4)*(Z2' * Z2)*((eps20^2)^(-1/4)) +  (-1/4)*((Z2' * Z2).^2)*((eps20^2)^(-5/4)) ;
    else
       S2 = ( (Z2' * Z2)^(3/4));        
    end
    
    % ALPHA1 derivative used in ALPHA2_HAT
    A1_dot = (ALPHA1 - last_A1)/tstep;
    last_A1 = ALPHA1;    
    
    % Calculate control signal
    AH2_A       = ( (0.5^(3/4))*a2 )*( (Z2 / (Z2' * Z2))*S2 );
    AH2_B       = ( (0.5^2)*b2) * ((Z2*(Z2' * Z2)           ));
    ALPHA2_HAT  = ( -(A1_dot) + AH2_A + AH2_B );
    g2          = inv(G2);
    CTRL        = -g2 * ( (Z2 .* (ALPHA2_HAT.^2)) ./ ( sqrt (((Z2.^2).*(ALPHA2_HAT.^2) + eps2^2)) ) + (Z2/(Z2'*Z2))*ETA_OMEGA'*g1*Z2 + F2 );
%   CTRL        = -g2 * ( (Z2 .* (ALPHA2_HAT.^2)) ./ ( sqrt (((Z2.^2).*(ALPHA2_HAT.^2) + eps2^2)) ) + (G1 * ETA_OMEGA) +F2 );  

%Function outputs
xErr    = [Z1(1) ; KH(1) ; -KL(1)];   % error and BLF limits
yErr    = [Z1(2) ; KH(2) ; -KL(2)];   % error and BLF limits
hErr    = [Z1(3) ; KH(3) ; -KL(3)];   % error and BLF limits
test1   = Z1 ;                        % test output
test2   = [tmax, a1, a2, b1, b2, eps1, eps2, eps10, eps20]';
u       = CTRL;


%%[2022.02.23.Wed] Changed Functions from v1.2(correcting for elementwise to matrix functions)

%     % Switched Term 1st step S1
%     if mETA < eps10
%         %test%S1 = ( (ETA.^2).^(3/4)); 
%         S1 = (5/4)*(ETA.^2)*((eps10^2)^(-1/4)) +  (-1/4)*((ETA.^2).^2)*((eps10^2)^(-5/4)) ;
%     else
%        S1 = ( (ETA.^2).^(3/4));        
%     end

%     % Calculate ALPHA1 virtual control for step 2
%     ALPHA1_HAT  = -(OMEGA.*Xd_dot) + ( ((0.5^(3/4)).*a1).*((ETA ./ (ETA.^2)).*S1) ) + ( ((0.5^2).*b1).*((ETA.*(ETA.^2))) );
%     ALPHA1_BAR  = diag([1/OMEGA(1) 1/OMEGA(2) 1/OMEGA(3)])*ALPHA1_HAT;
%     nA1B        = norm(ALPHA1_BAR);
%     ETA_OMEGA   = ETA .* OMEGA;
%     nETA_OMEGA  = norm(ETA_OMEGA);
%     g1          = inv(G1);

    % wrong sqrt in denom of ALPHA1 below
%   ALPHA1      = -g1 * (( ETA_OMEGA*((nA1B)^2) ) ./ (sqrt( (nETA_OMEGA)^2)*((nA1B)^2) + eps1^2  ));
